simulink model "model1"  (R2020a)
settings: Solver=FixedStepAuto  StartTime=0.0  StopTime=3600  FixedStep=1  RelTol=1e-3
libraries: fuzblock x3
settings Model: Creator=ji180550d  LastModifiedBy=ji180550d

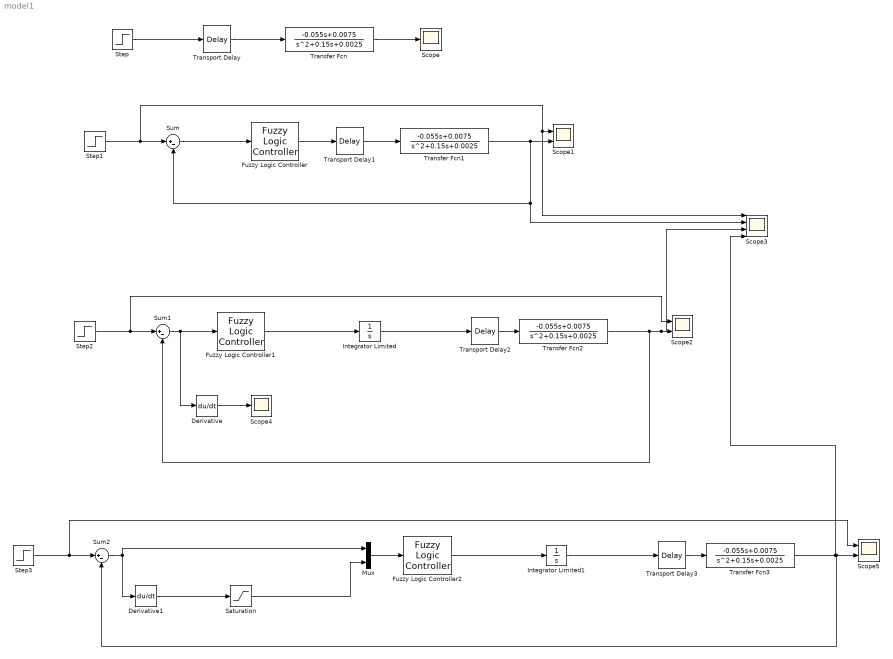
== system model1 ==
  Derivative : Derivative
  Derivative1 : Derivative
  Fuzzy Logic Controller : fuzblock/Fuzzy Logic  Controller  FIS='resenje1.fis'  OutputSampleNumber=101  DataType=double  FuzzifiedInputs=off  RuleFiringStrengths=off  RuleOutputs=off  AggregatedOutputs=off  SimulateUsing=Interpreted execution  OutOfRangeInputValueMessage=warning  NoRuleFiredMessage=warning  EmptyOutputFuzzySetMessage=warning
  Fuzzy Logic Controller1 : fuzblock/Fuzzy Logic  Controller  FIS='resenje2.fis'  OutputSampleNumber=101  DataType=double  FuzzifiedInputs=off  RuleFiringStrengths=off  RuleOutputs=off  AggregatedOutputs=off  SimulateUsing=Interpreted execution  OutOfRangeInputValueMessage=warning  NoRuleFiredMessage=warning  EmptyOutputFuzzySetMessage=warning
  Fuzzy Logic Controller2 : fuzblock/Fuzzy Logic  Controller  FIS='resenje3.fis'  OutputSampleNumber=101  DataType=double  FuzzifiedInputs=off  RuleFiringStrengths=off  RuleOutputs=off  AggregatedOutputs=off  SimulateUsing=Interpreted execution  OutOfRangeInputValueMessage=warning  NoRuleFiredMessage=warning  EmptyOutputFuzzySetMessage=warning
  Integrator Limited : Integrator  LimitOutput=on  UpperSaturationLimit=1.2  LowerSaturationLimit=-1.2
  Integrator Limited1 : Integrator  LimitOutput=on  UpperSaturationLimit=1.2  LowerSaturationLimit=-1.2
  Mux : Mux  Inputs=2
  Saturation : Saturate  UpperLimit=0.18  LowerLimit=-0.18
  Scope : Scope
  Scope1 : Scope  NumInputPorts=2
  Scope2 : Scope  NumInputPorts=2
  Scope3 : Scope  NumInputPorts=4
  Scope4 : Scope
  Scope5 : Scope  NumInputPorts=2
  Step{,1..3} (4 alike) : Step  Time=1000  Before=2  After=-2  SampleTime=0
  Sum : Sum  Inputs=|+-
  Sum1 : Sum  Inputs=|+-
  Sum2 : Sum  Inputs=|+-
  Transfer Fcn{,1..3} (4 alike) : TransferFcn  Numerator=[-0.055 0.0075]  Denominator=[1 0.15 0.0025]
  Transport Delay{,1..3} (4 alike) : TransportDelay  DelayTime=3.6
  wires:
  Step/1 -> Transport Delay/1
  Transport Delay/1 -> Transfer Fcn/1
  Transfer Fcn/1 -> Scope/1
  Transport Delay1/1 -> Transfer Fcn1/1
  Fuzzy Logic Controller/1 -> Transport Delay1/1
  Sum/1 -> Fuzzy Logic Controller/1
  Sum1/1 -> Derivative/1, Fuzzy Logic Controller1/1
  Transport Delay2/1 -> Transfer Fcn2/1
  Step2/1 -> Scope2/1, Sum1/1
  Integrator Limited/1 -> Transport Delay2/1
  Fuzzy Logic Controller1/1 -> Integrator Limited/1
  Step1/1 -> Scope3/1, Scope1/1, Sum/1
  Transfer Fcn1/1 -> Scope1/2, Scope3/2, Sum/2
  Transfer Fcn2/1 -> Scope3/3, Scope2/2, Sum1/2
  Derivative/1 -> Scope4/1
  Integrator Limited1/1 -> Transport Delay3/1
  Fuzzy Logic Controller2/1 -> Integrator Limited1/1
  Derivative1/1 -> Saturation/1
  Transport Delay3/1 -> Transfer Fcn3/1
  Sum2/1 -> Derivative1/1, Mux/1
  Step3/1 -> Scope5/1, Sum2/1
  Mux/1 -> Fuzzy Logic Controller2/1
  Saturation/1 -> Mux/2
  Transfer Fcn3/1 -> Scope5/2, Sum2/2, Scope3/4
